simulink model "DSM1ORDER20250930"  (R2024b)
settings: Solver=VariableStepAuto  StartTime=0.0  StopTime=1  RelTol=1e-3
settings Model: Creator=gjp88  LastModifiedBy=gjp88

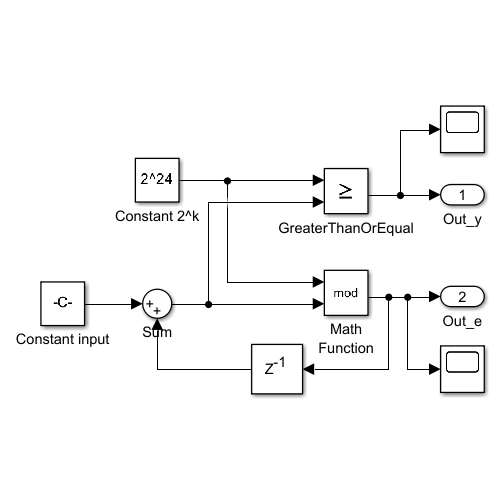
[thumbnail: Simulink's stored preview of the top-level diagram]
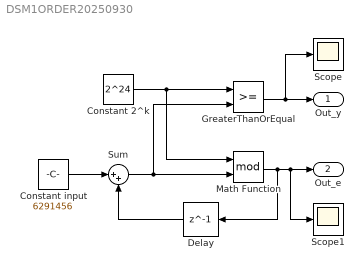
== system DSM1ORDER20250930 ==
  Constant 2^k : Constant  Value=2^24  SampleTime=0
  Constant input : Constant  Value=6291456  SampleTime=0
  Delay : Delay  DelayLength=1  InitialCondition=0
  GreaterThanOrEqual : RelationalOperator  OutDataTypeStr=boolean  RndMeth=Simplest  InputSameDT=off
  Math Function : Math  Operator=mod
  Scope : Scope
  Scope1 : Scope
  Sum : Sum  Inputs=|++
  Out_y : Outport
  Out_e : Outport  Port=2
  wires:
  Constant 2^k/1 -> Math Function/1, GreaterThanOrEqual/1
  GreaterThanOrEqual/1 -> Scope/1, Out_y/1
  Math Function/1 -> Delay/1, Scope1/1, Out_e/1
  Delay/1 -> Sum/2
  Sum/1 -> GreaterThanOrEqual/2, Math Function/2
  Constant input/1 -> Sum/1
